simulink model "SimPIDlatdir2020b"  (R2020b)
settings: Solver=VariableStepAuto  StartTime=0.0  StopTime=10  RelTol=1e-3
values from neighbouring files (symbols this model uses):
  g_p_ail = tf(modelo(2,1))    [latdirPID.m]
  g_p_rud = tf(modelo(2,2))    [latdirPID.m]
  g_phi_ail = tf(modelo(4,1))    [latdirPID.m]
  g_phi_rud = tf(modelo(4,2))    [latdirPID.m]
  g_psi_ail = tf(modelo(5,2))    [latdirPID.m]
  g_psi_rud = tf(modelo(5,2))    [latdirPID.m]
  g_r_ail = tf(modelo(3,1))    [latdirPID.m]
  g_r_rud = tf(modelo(3,2))    [latdirPID.m]
  Kd_a = 2    [latdirPID.m]
  Kd_r = 2    [latdirPID.m]
  Ki_a = 0.002    [latdirPID.m]
  Ki_r = 0.002    [latdirPID.m]
  Kp_a = 7    [latdirPID.m]
  Kp_r = 7    [latdirPID.m]
libraries: pid_lib x16, simulink x4
(part 2 of 2)

== system SimPIDlatdir2020b/LatDir Ruido/Pos modelo/CAS_Yaw ==
  Ail : Inport
  Rud : Inport  Port=2
  CAS_ail : pid_lib/PID Controller  Controller=PI  Form=Parallel  TimeDomain=Continuous-time  UseExternalTs=off  SampleTime=-1  IntegratorMethod=Forward Euler  FilterMethod=Forward Euler  ControllerParametersSource=internal  P=Kp_a  I=Ki_a  D=0  N=100  UseFilter=on  TunerSelectOption=Transfer Function Based (PID Tuner App)  InitialConditionSource=internal  InitialConditionForIntegrator=0  InitialConditionForFilter=0  DifferentiatorICPrevScaledInput=0  ExternalReset=none  TrackingMode=off  Kt=1  LimitOutput=off  SatLimitsSource=internal  UpperSaturationLimit=inf  LowerSaturationLimit=-inf  LinearizeAsGain=on  AntiWindupMode=none  Kb=1  POutMin=[]  POutMax=[]  IOutMin=[]  IOutMax=[]  DOutMin=[]  DOutMax=[]  NOutMin=[]  NOutMax=[]  SumOutMin=[]  SumOutMax=[]  SaturationOutMin=[]  SaturationOutMax=[]  PParamMin=[]  PParamMax=[]  IParamMin=[]  IParamMax=[]  DParamMin=[]  DParamMax=[]  NParamMin=[]  NParamMax=[]  KbParamMin=[]  KbParamMax=[]  KtParamMin=[]  KtParamMax=[]  KbOutMin=[]  KbOutMax=[]  KtOutMin=[]  KtOutMax=[]  IntegratorOutMin=[]  IntegratorOutMax=[]  FilterOutMin=[]  FilterOutMax=[]  SumI1OutMin=[]  SumI1OutMax=[]  SumI2OutMin=[]  SumI2OutMax=[]  SumI3OutMin=[]  SumI3OutMax=[]  SumI4OutMin=[]  SumI4OutMax=[]  SumDOutMin=[]  SumDOutMax=[]  DifferentiatorOutMin=[]  DifferentiatorOutMax=[]  FilterDiffOutCoefMin=[]  FilterDiffOutCoefMax=[]  ReciprocalOutMin=[]  ReciprocalOutMax=[]  SumDenOutMin=[]  SumDenOutMax=[]  SumNumOutMin=[]  SumNumOutMax=[]  DivideOutMin=[]  DivideOutMax=[]  UdiffTsProdOutMin=[]  UdiffTsProdOutMax=[]  NTsProdOutMin=[]  NTsProdOutMax=[]  UintegralTsProdOutMin=[]  UintegralTsProdOutMax=[]  UngainTsProdOutMin=[]  UngainTsProdOutMax=[]  IntegratorContinuousStateAttributes=''  IntegratorStateMustResolveToSignalObject=off  IntegratorRTWStateStorageClass=Auto  FilterContinuousStateAttributes=''  FilterStateMustResolveToSignalObject=off  FilterRTWStateStorageClass=Auto  ParallelPVariant=InternalParameters  IdealPVariant=Disabled  IVariant=InternalParameters  DVariant=Disabled  IntegratorVariant=Continuous  SatVariant=Disabled  AWVariant=Passthrough  PCopyVariant=Disabled  TRVariant=Disabled  FdbkBlocksVariant=Forward  IdealPFdbkVariant=Disabled  SatFdbkVariant=Disabled  DerivativeFilterVariant=Disabled  NVariant=Disabled  NCopyVariant=Disabled_SignalSpec  FilterICVariant=Disabled  IntegratorICVariant=InternalICs  ExternalResetVariant=Disabled  TRSumVariant=Passthrough  SumFdbkVariant=Disabled  SumVariant=Sum_PI  TsampFilterVariant=InternalTs  TsampNgainVariant=Passthrough  TsampIntegralVariant=Passthrough  ExternalSaturationOutDataTypeStr=Inherit: Same as second input
  CAS_rud : pid_lib/PID Controller  Controller=PI  Form=Parallel  TimeDomain=Continuous-time  UseExternalTs=off  SampleTime=-1  IntegratorMethod=Forward Euler  FilterMethod=Forward Euler  ControllerParametersSource=internal  P=Kp_r  I=Ki_r  D=0  N=100  UseFilter=on  TunerSelectOption=Transfer Function Based (PID Tuner App)  InitialConditionSource=internal  InitialConditionForIntegrator=0  InitialConditionForFilter=0  DifferentiatorICPrevScaledInput=0  ExternalReset=none  TrackingMode=off  Kt=1  LimitOutput=off  SatLimitsSource=internal  UpperSaturationLimit=inf  LowerSaturationLimit=-inf  LinearizeAsGain=on  AntiWindupMode=none  Kb=1  POutMin=[]  POutMax=[]  IOutMin=[]  IOutMax=[]  DOutMin=[]  DOutMax=[]  NOutMin=[]  NOutMax=[]  SumOutMin=[]  SumOutMax=[]  SaturationOutMin=[]  SaturationOutMax=[]  PParamMin=[]  PParamMax=[]  IParamMin=[]  IParamMax=[]  DParamMin=[]  DParamMax=[]  NParamMin=[]  NParamMax=[]  KbParamMin=[]  KbParamMax=[]  KtParamMin=[]  KtParamMax=[]  KbOutMin=[]  KbOutMax=[]  KtOutMin=[]  KtOutMax=[]  IntegratorOutMin=[]  IntegratorOutMax=[]  FilterOutMin=[]  FilterOutMax=[]  SumI1OutMin=[]  SumI1OutMax=[]  SumI2OutMin=[]  SumI2OutMax=[]  SumI3OutMin=[]  SumI3OutMax=[]  SumI4OutMin=[]  SumI4OutMax=[]  SumDOutMin=[]  SumDOutMax=[]  DifferentiatorOutMin=[]  DifferentiatorOutMax=[]  FilterDiffOutCoefMin=[]  FilterDiffOutCoefMax=[]  ReciprocalOutMin=[]  ReciprocalOutMax=[]  SumDenOutMin=[]  SumDenOutMax=[]  SumNumOutMin=[]  SumNumOutMax=[]  DivideOutMin=[]  DivideOutMax=[]  UdiffTsProdOutMin=[]  UdiffTsProdOutMax=[]  NTsProdOutMin=[]  NTsProdOutMax=[]  UintegralTsProdOutMin=[]  UintegralTsProdOutMax=[]  UngainTsProdOutMin=[]  UngainTsProdOutMax=[]  IntegratorContinuousStateAttributes=''  IntegratorStateMustResolveToSignalObject=off  IntegratorRTWStateStorageClass=Auto  FilterContinuousStateAttributes=''  FilterStateMustResolveToSignalObject=off  FilterRTWStateStorageClass=Auto  ParallelPVariant=InternalParameters  IdealPVariant=Disabled  IVariant=InternalParameters  DVariant=Disabled  IntegratorVariant=Continuous  SatVariant=Disabled  AWVariant=Passthrough  PCopyVariant=Disabled  TRVariant=Disabled  FdbkBlocksVariant=Forward  IdealPFdbkVariant=Disabled  SatFdbkVariant=Disabled  DerivativeFilterVariant=Disabled  NVariant=Disabled  NCopyVariant=Disabled_SignalSpec  FilterICVariant=Disabled  IntegratorICVariant=InternalICs  ExternalResetVariant=Disabled  TRSumVariant=Passthrough  SumFdbkVariant=Disabled  SumVariant=Sum_PI  TsampFilterVariant=InternalTs  TsampNgainVariant=Passthrough  TsampIntegralVariant=Passthrough  ExternalSaturationOutDataTypeStr=Inherit: Same as second input
  SAS : Subsystem
  Sum : Sum  Inputs=-+|
  Sum1 : Sum  Inputs=|+-
  Psi : Outport
  wires:
  Sum1/1 -> CAS_rud/1
  Rud/1 -> Sum1/1
  Sum/1 -> CAS_ail/1
  CAS_rud/1 -> SAS/2("rud ")
  SAS/1(Psi) -> Psi/1, Sum1/2, Sum/1
  CAS_ail/1 -> SAS/1(ail)
  Ail/1 -> Sum/2

== system SimPIDlatdir2020b/LatDir/Pos integrada/CAS_Roll2/SAS ==
  note: Se realimenta la velocidad del ángulo phi como contribución de
      | cada uno de los actuadores.
  ail : Inport
  "rud " : Inport  Port=2
  Kd_ail : Gain  Gain=Kd_a
  Kd_rud : Gain  Gain=Kd_r
  Roll : Subsystem
  Sum : Sum  Inputs=-+|
  Sum1 : Sum  Inputs=|+-
  Phi : Outport
  wires:
  Sum1/1 -> Roll/2("rud ")
  Sum/1 -> Roll/1(ail)
  Kd_rud/1 -> Sum1/2
  Kd_ail/1 -> Sum/1
  ail/1 -> Sum/2
  "rud "/1 -> Sum1/1
  Roll/1(Phi) -> Phi/1
  Roll/2(Phi_dot) -> Kd_ail/1, Kd_rud/1

== system SimPIDlatdir2020b/LatDir/Pos integrada/CAS_Yaw2/SAS ==
  note: Se realimenta la velocidad del ángulo phi como contribución de
      | cada uno de los actuadores.
  ail : Inport
  "rud " : Inport  Port=2
  Kd_ail : Gain  Gain=Kd_a
  Kd_rud : Gain  Gain=Kd_r
  Sum : Sum  Inputs=-+|
  Sum1 : Sum  Inputs=|+-
  Yaw : Subsystem
  Psi : Outport
  wires:
  Yaw/2(Psi_dot) -> Kd_ail/1, Kd_rud/1
  Yaw/1(Psi) -> Psi/1
  "rud "/1 -> Sum1/1
  ail/1 -> Sum/2
  Kd_ail/1 -> Sum/1
  Kd_rud/1 -> Sum1/2
  Sum/1 -> Yaw/1(ail)
  Sum1/1 -> Yaw/2("rud ")

== system SimPIDlatdir2020b/LatDir/Pos modelo/CAS_Roll/SAS ==
  note: Se realimenta la velocidad del ángulo phi como contribución de
      | cada uno de los actuadores.
  ail : Inport
  "rud " : Inport  Port=2
  Kd_ail : Gain  Gain=Kd_a
  Kd_rud : Gain  Gain=Kd_r
  Roll : Subsystem
  Sum : Sum  Inputs=-+|
  Sum1 : Sum  Inputs=|+-
  Phi : Outport
  wires:
  Roll/2(Phi_dot) -> Kd_rud/1, Kd_ail/1
  Roll/1(Phi) -> Phi/1
  "rud "/1 -> Sum1/1
  ail/1 -> Sum/2
  Kd_ail/1 -> Sum/1
  Kd_rud/1 -> Sum1/2
  Sum/1 -> Roll/1(ail)
  Sum1/1 -> Roll/2("rud ")

== system SimPIDlatdir2020b/LatDir/Pos modelo/CAS_Yaw/SAS ==
  note: Se realimenta la velocidad del ángulo phi como contribución de
      | cada uno de los actuadores.
  ail : Inport
  "rud " : Inport  Port=2
  Kd_ail : Gain  Gain=Kd_a
  Kd_rud : Gain  Gain=Kd_r
  Sum : Sum  Inputs=-+|
  Sum1 : Sum  Inputs=|+-
  Yaw : Subsystem
  Psi : Outport
  wires:
  Sum1/1 -> Yaw/2("rud ")
  Sum/1 -> Yaw/1(ail)
  Kd_rud/1 -> Sum1/2
  Kd_ail/1 -> Sum/1
  ail/1 -> Sum/2
  "rud "/1 -> Sum1/1
  Yaw/1(Psi) -> Psi/1
  Yaw/2(Psi_dot) -> Kd_rud/1, Kd_ail/1

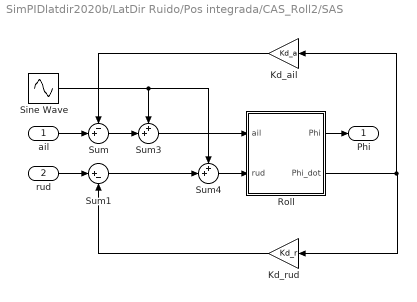
== system SimPIDlatdir2020b/LatDir Ruido/Pos integrada/CAS_Roll2/SAS ==
  ail : Inport
  "rud " : Inport  Port=2
  Kd_ail : Gain  Gain=Kd_a
  Kd_rud : Gain  Gain=Kd_r
  Roll : Subsystem
  Sine Wave : Sin  SampleTime=0
  Sum : Sum  Inputs=-+|
  Sum1 : Sum  Inputs=|+-
  Sum3 : Sum  Inputs=++|
  Sum4 : Sum  Inputs=++|
  Phi : Outport
  wires:
  Roll/1(Phi) -> Phi/1
  "rud "/1 -> Sum1/1
  ail/1 -> Sum/2
  Kd_ail/1 -> Sum/1
  Kd_rud/1 -> Sum1/2
  Sum1/1 -> Sum4/2
  Sum4/1 -> Roll/2("rud ")
  Sum/1 -> Sum3/2
  Sum3/1 -> Roll/1(ail)
  Sine Wave/1 -> Sum4/1, Sum3/1
  Roll/2(Phi_dot) -> Kd_ail/1, Kd_rud/1

== system SimPIDlatdir2020b/LatDir Ruido/Pos integrada/CAS_Yaw2/SAS ==
  ail : Inport
  "rud " : Inport  Port=2
  Kd_ail : Gain  Gain=Kd_a
  Kd_rud : Gain  Gain=Kd_r
  Sum : Sum  Inputs=-+|
  Sum1 : Sum  Inputs=|+-
  Yaw : Subsystem
  Psi : Outport
  wires:
  Sum1/1 -> Yaw/2("rud ")
  Sum/1 -> Yaw/1(ail)
  Kd_rud/1 -> Sum1/2
  Kd_ail/1 -> Sum/1
  ail/1 -> Sum/2
  "rud "/1 -> Sum1/1
  Yaw/1(Psi) -> Psi/1
  Yaw/2(Psi_dot) -> Kd_rud/1, Kd_ail/1

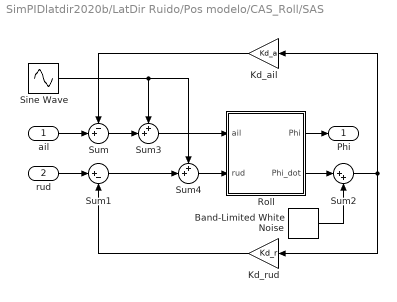
== system SimPIDlatdir2020b/LatDir Ruido/Pos modelo/CAS_Roll/SAS ==
  ail : Inport
  "rud " : Inport  Port=2
  Band-Limited White Noise : simulink/Sources/Band-Limited White Noise  Cov=[0.001]  Ts=0.1  seed=[23341]
  Kd_ail : Gain  Gain=Kd_a
  Kd_rud : Gain  Gain=Kd_r
  Roll : Subsystem
  Sine Wave : Sin  Frequency=12*pi  SampleTime=0
  Sum : Sum  Inputs=-+|
  Sum1 : Sum  Inputs=|+-
  Sum2 : Sum  Inputs=|++
  Sum3 : Sum  Inputs=++|
  Sum4 : Sum  Inputs=++|
  Phi : Outport
  wires:
  Kd_rud/1 -> Sum1/2
  Kd_ail/1 -> Sum/1
  ail/1 -> Sum/2
  "rud "/1 -> Sum1/1
  Roll/1(Phi) -> Phi/1
  Roll/2(Phi_dot) -> Sum2/1
  Sum2/1 -> Kd_rud/1, Kd_ail/1
  Band-Limited White Noise/1 -> Sum2/2
  Sum/1 -> Sum3/2
  Sum3/1 -> Roll/1(ail)
  Sum4/1 -> Roll/2("rud ")
  Sum1/1 -> Sum4/2
  Sine Wave/1 -> Sum4/1, Sum3/1

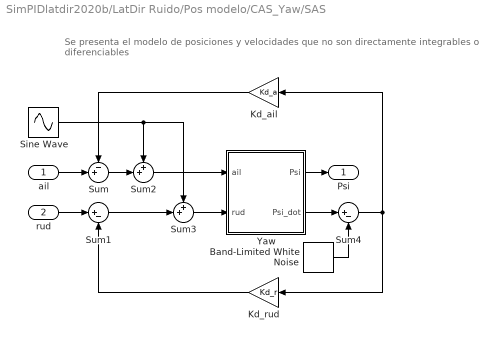
== system SimPIDlatdir2020b/LatDir Ruido/Pos modelo/CAS_Yaw/SAS ==
  note: Se presenta el modelo de posiciones y velocidades que no son directamente integrables o diferenciables
  ail : Inport
  "rud " : Inport  Port=2
  Band-Limited White Noise : simulink/Sources/Band-Limited White Noise  Cov=0.001  Ts=0.1  seed=[23341]
  Kd_ail : Gain  Gain=Kd_a
  Kd_rud : Gain  Gain=Kd_r
  Sine Wave : Sin  Frequency=12*pi  SampleTime=0
  Sum : Sum  Inputs=-+|
  Sum1 : Sum  Inputs=|+-
  Sum2 : Sum  Inputs=++|
  Sum3 : Sum  Inputs=++|
  Sum4 : Sum  Inputs=|+-
  Yaw : Subsystem
  Psi : Outport
  wires:
  Yaw/1(Psi) -> Psi/1
  "rud "/1 -> Sum1/1
  ail/1 -> Sum/2
  Kd_ail/1 -> Sum/1
  Kd_rud/1 -> Sum1/2
  Sum/1 -> Sum2/2
  Sum2/1 -> Yaw/1(ail)
  Sum3/1 -> Yaw/2("rud ")
  Sum1/1 -> Sum3/2
  Sine Wave/1 -> Sum3/1, Sum2/1
  Yaw/2(Psi_dot) -> Sum4/1
  Sum4/1 -> Kd_ail/1, Kd_rud/1
  Band-Limited White Noise/1 -> Sum4/2

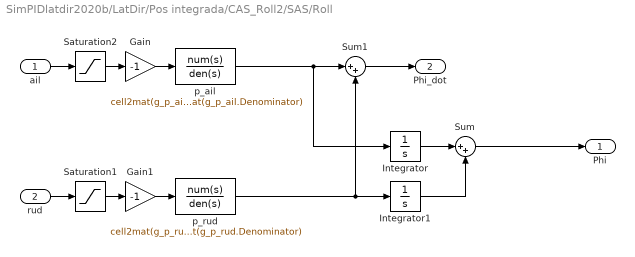
== system SimPIDlatdir2020b/LatDir/Pos integrada/CAS_Roll2/SAS/Roll ==
  ail : Inport
  "rud " : Inport  Port=2
  Gain : Gain  Gain=-1
  Gain1 : Gain  Gain=-1
  Integrator : Integrator
  Integrator1 : Integrator
  Saturation1 : Saturate  UpperLimit=30  LowerLimit=-30
  Saturation2 : Saturate  UpperLimit=30  LowerLimit=-30
  Sum : Sum  Inputs=|++
  Sum1 : Sum  Inputs=|++
  p_ail : TransferFcn  Numerator=cell2mat(g_p_ail.Numerator)  Denominator=cell2mat(g_p_ail.Denominator)
  p_rud : TransferFcn  Numerator=cell2mat(g_p_rud.Numerator)  Denominator=cell2mat(g_p_rud.Denominator)
  Phi : Outport
  Phi_dot : Outport  Port=2
  wires:
  "rud "/1 -> Saturation1/1
  Gain1/1 -> p_rud/1
  Gain/1 -> p_ail/1
  Sum/1 -> Phi/1
  Sum1/1 -> Phi_dot/1
  p_ail/1 -> Integrator/1, Sum1/1
  p_rud/1 -> Sum1/2, Integrator1/1
  ail/1 -> Saturation2/1
  Integrator/1 -> Sum/1
  Integrator1/1 -> Sum/2
  Saturation2/1 -> Gain/1
  Saturation1/1 -> Gain1/1

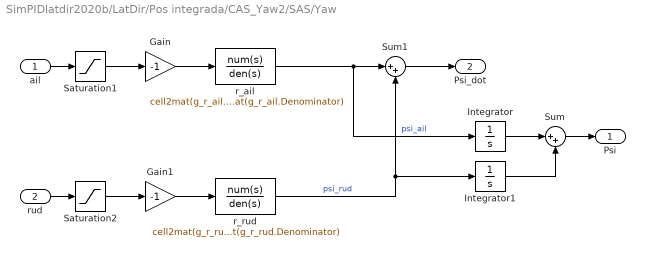
== system SimPIDlatdir2020b/LatDir/Pos integrada/CAS_Yaw2/SAS/Yaw ==
  ail : Inport
  "rud " : Inport  Port=2
  Gain : Gain  Gain=-1
  Gain1 : Gain  Gain=-1
  Integrator : Integrator
  Integrator1 : Integrator
  Saturation1 : Saturate  UpperLimit=30  LowerLimit=-30
  Saturation2 : Saturate  UpperLimit=30  LowerLimit=-30
  Sum : Sum  Inputs=|++
  Sum1 : Sum  Inputs=|++
  r_ail : TransferFcn  Numerator=cell2mat(g_r_ail.Numerator)  Denominator=cell2mat(g_r_ail.Denominator)
  r_rud : TransferFcn  Numerator=cell2mat(g_r_rud.Numerator)  Denominator=cell2mat(g_r_rud.Denominator)
  Psi : Outport
  Psi_dot : Outport  Port=2
  wires:
  "rud "/1 -> Saturation2/1
  ail/1 -> Saturation1/1
  r_rud/1 -> Integrator1/1, Sum1/2  "psi_rud"
  r_ail/1 -> Integrator/1, Sum1/1  "psi_ail"
  Sum1/1 -> Psi_dot/1
  Sum/1 -> Psi/1
  Integrator1/1 -> Sum/2
  Integrator/1 -> Sum/1
  Saturation1/1 -> Gain/1
  Saturation2/1 -> Gain1/1
  Gain/1 -> r_ail/1
  Gain1/1 -> r_rud/1

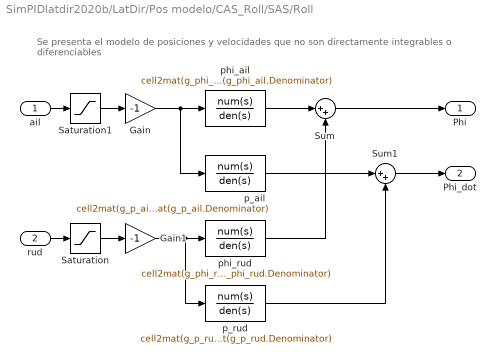
== system SimPIDlatdir2020b/LatDir/Pos modelo/CAS_Roll/SAS/Roll ==
  note: Se presenta el modelo de posiciones y velocidades que no son directamente integrables o diferenciables
  ail : Inport
  "rud " : Inport  Port=2
  Gain : Gain  Gain=-1
  Gain1 : Gain  Gain=-1
  Saturation : Saturate  UpperLimit=30  LowerLimit=-30
  Saturation1 : Saturate  UpperLimit=30  LowerLimit=-30
  Sum : Sum  Inputs=|++
  Sum1 : Sum  Inputs=|++
  p_ail : TransferFcn  Numerator=cell2mat(g_p_ail.Numerator)  Denominator=cell2mat(g_p_ail.Denominator)
  p_rud : TransferFcn  Numerator=cell2mat(g_p_rud.Numerator)  Denominator=cell2mat(g_p_rud.Denominator)
  phi_ail : TransferFcn  Numerator=cell2mat(g_phi_ail.Numerator)  Denominator=cell2mat(g_phi_ail.Denominator)
  phi_rud : TransferFcn  Numerator=cell2mat(g_phi_rud.Numerator)  Denominator=cell2mat(g_phi_rud.Denominator)
  Phi : Outport
  Phi_dot : Outport  Port=2
  wires:
  ail/1 -> Saturation1/1
  p_rud/1 -> Sum1/2
  p_ail/1 -> Sum1/1
  phi_ail/1 -> Sum/1
  Sum1/1 -> Phi_dot/1
  phi_rud/1 -> Sum/2
  Sum/1 -> Phi/1
  Gain/1 -> p_ail/1, phi_ail/1
  Gain1/1 -> p_rud/1, phi_rud/1
  "rud "/1 -> Saturation/1
  Saturation/1 -> Gain1/1
  Saturation1/1 -> Gain/1

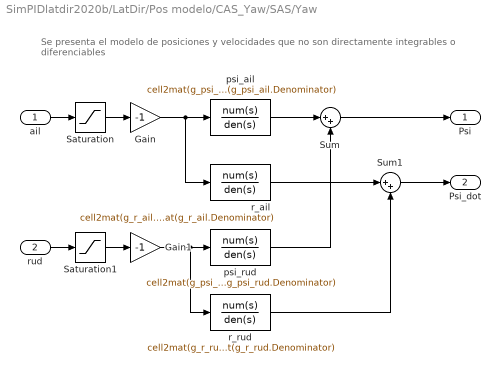
== system SimPIDlatdir2020b/LatDir/Pos modelo/CAS_Yaw/SAS/Yaw ==
  note: Se presenta el modelo de posiciones y velocidades que no son directamente integrables o diferenciables
  ail : Inport
  "rud " : Inport  Port=2
  Gain : Gain  Gain=-1
  Gain1 : Gain  Gain=-1
  Saturation : Saturate  UpperLimit=30  LowerLimit=-30
  Saturation1 : Saturate  UpperLimit=30  LowerLimit=-30
  Sum : Sum  Inputs=|++
  Sum1 : Sum  Inputs=|++
  psi_ail : TransferFcn  Numerator=cell2mat(g_psi_ail.Numerator)  Denominator=cell2mat(g_psi_ail.Denominator)
  psi_rud : TransferFcn  Numerator=cell2mat(g_psi_rud.Numerator)  Denominator=cell2mat(g_psi_rud.Denominator)
  r_ail : TransferFcn  Numerator=cell2mat(g_r_ail.Numerator)  Denominator=cell2mat(g_r_ail.Denominator)
  r_rud : TransferFcn  Numerator=cell2mat(g_r_rud.Numerator)  Denominator=cell2mat(g_r_rud.Denominator)
  Psi : Outport
  Psi_dot : Outport  Port=2
  wires:
  Sum/1 -> Psi/1
  psi_rud/1 -> Sum/2
  Sum1/1 -> Psi_dot/1
  psi_ail/1 -> Sum/1
  r_ail/1 -> Sum1/1
  r_rud/1 -> Sum1/2
  ail/1 -> Saturation/1
  "rud "/1 -> Saturation1/1
  Gain/1 -> r_ail/1, psi_ail/1
  Gain1/1 -> r_rud/1, psi_rud/1
  Saturation/1 -> Gain/1
  Saturation1/1 -> Gain1/1

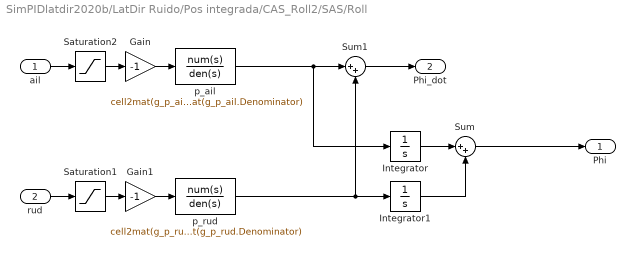
== system SimPIDlatdir2020b/LatDir Ruido/Pos integrada/CAS_Roll2/SAS/Roll ==
  ail : Inport
  "rud " : Inport  Port=2
  Gain : Gain  Gain=-1
  Gain1 : Gain  Gain=-1
  Integrator : Integrator
  Integrator1 : Integrator
  Saturation1 : Saturate  UpperLimit=30  LowerLimit=-30
  Saturation2 : Saturate  UpperLimit=30  LowerLimit=-30
  Sum : Sum  Inputs=|++
  Sum1 : Sum  Inputs=|++
  p_ail : TransferFcn  Numerator=cell2mat(g_p_ail.Numerator)  Denominator=cell2mat(g_p_ail.Denominator)
  p_rud : TransferFcn  Numerator=cell2mat(g_p_rud.Numerator)  Denominator=cell2mat(g_p_rud.Denominator)
  Phi : Outport
  Phi_dot : Outport  Port=2
  wires:
  Saturation1/1 -> Gain1/1
  Saturation2/1 -> Gain/1
  Integrator1/1 -> Sum/2
  Integrator/1 -> Sum/1
  ail/1 -> Saturation2/1
  p_rud/1 -> Integrator1/1, Sum1/2
  p_ail/1 -> Sum1/1, Integrator/1
  Sum1/1 -> Phi_dot/1
  Sum/1 -> Phi/1
  Gain/1 -> p_ail/1
  Gain1/1 -> p_rud/1
  "rud "/1 -> Saturation1/1

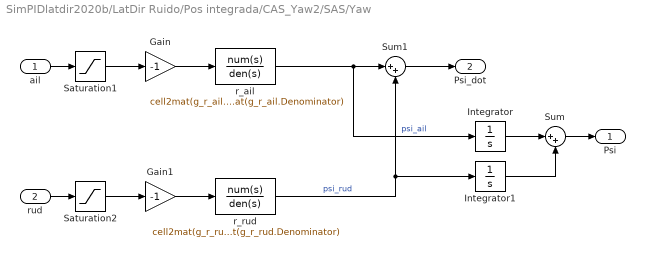
== system SimPIDlatdir2020b/LatDir Ruido/Pos integrada/CAS_Yaw2/SAS/Yaw ==
  ail : Inport
  "rud " : Inport  Port=2
  Gain : Gain  Gain=-1
  Gain1 : Gain  Gain=-1
  Integrator : Integrator
  Integrator1 : Integrator
  Saturation1 : Saturate  UpperLimit=30  LowerLimit=-30
  Saturation2 : Saturate  UpperLimit=30  LowerLimit=-30
  Sum : Sum  Inputs=|++
  Sum1 : Sum  Inputs=|++
  r_ail : TransferFcn  Numerator=cell2mat(g_r_ail.Numerator)  Denominator=cell2mat(g_r_ail.Denominator)
  r_rud : TransferFcn  Numerator=cell2mat(g_r_rud.Numerator)  Denominator=cell2mat(g_r_rud.Denominator)
  Psi : Outport
  Psi_dot : Outport  Port=2
  wires:
  Gain1/1 -> r_rud/1
  Gain/1 -> r_ail/1
  Saturation2/1 -> Gain1/1
  Saturation1/1 -> Gain/1
  Integrator/1 -> Sum/1
  Integrator1/1 -> Sum/2
  Sum/1 -> Psi/1
  Sum1/1 -> Psi_dot/1
  r_ail/1 -> Sum1/1, Integrator/1  "psi_ail"
  r_rud/1 -> Sum1/2, Integrator1/1  "psi_rud"
  ail/1 -> Saturation1/1
  "rud "/1 -> Saturation2/1

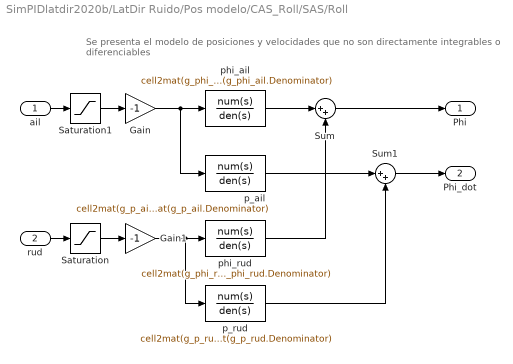
== system SimPIDlatdir2020b/LatDir Ruido/Pos modelo/CAS_Roll/SAS/Roll ==
  note: Se presenta el modelo de posiciones y velocidades que no son directamente integrables o diferenciables
  ail : Inport
  "rud " : Inport  Port=2
  Gain : Gain  Gain=-1
  Gain1 : Gain  Gain=-1
  Saturation : Saturate  UpperLimit=30  LowerLimit=-30
  Saturation1 : Saturate  UpperLimit=30  LowerLimit=-30
  Sum : Sum  Inputs=|++
  Sum1 : Sum  Inputs=|++
  p_ail : TransferFcn  Numerator=cell2mat(g_p_ail.Numerator)  Denominator=cell2mat(g_p_ail.Denominator)
  p_rud : TransferFcn  Numerator=cell2mat(g_p_rud.Numerator)  Denominator=cell2mat(g_p_rud.Denominator)
  phi_ail : TransferFcn  Numerator=cell2mat(g_phi_ail.Numerator)  Denominator=cell2mat(g_phi_ail.Denominator)
  phi_rud : TransferFcn  Numerator=cell2mat(g_phi_rud.Numerator)  Denominator=cell2mat(g_phi_rud.Denominator)
  Phi : Outport
  Phi_dot : Outport  Port=2
  wires:
  Saturation1/1 -> Gain/1
  Saturation/1 -> Gain1/1
  "rud "/1 -> Saturation/1
  Gain1/1 -> phi_rud/1, p_rud/1
  Gain/1 -> phi_ail/1, p_ail/1
  Sum/1 -> Phi/1
  phi_rud/1 -> Sum/2
  Sum1/1 -> Phi_dot/1
  phi_ail/1 -> Sum/1
  p_ail/1 -> Sum1/1
  p_rud/1 -> Sum1/2
  ail/1 -> Saturation1/1

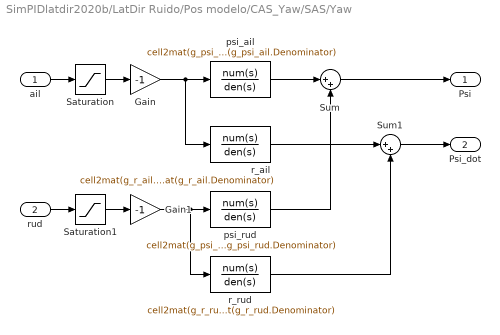
== system SimPIDlatdir2020b/LatDir Ruido/Pos modelo/CAS_Yaw/SAS/Yaw ==
  ail : Inport
  "rud " : Inport  Port=2
  Gain : Gain  Gain=-1
  Gain1 : Gain  Gain=-1
  Saturation : Saturate  UpperLimit=30  LowerLimit=-30
  Saturation1 : Saturate  UpperLimit=30  LowerLimit=-30
  Sum : Sum  Inputs=|++
  Sum1 : Sum  Inputs=|++
  psi_ail : TransferFcn  Numerator=cell2mat(g_psi_ail.Numerator)  Denominator=cell2mat(g_psi_ail.Denominator)
  psi_rud : TransferFcn  Numerator=cell2mat(g_psi_rud.Numerator)  Denominator=cell2mat(g_psi_rud.Denominator)
  r_ail : TransferFcn  Numerator=cell2mat(g_r_ail.Numerator)  Denominator=cell2mat(g_r_ail.Denominator)
  r_rud : TransferFcn  Numerator=cell2mat(g_r_rud.Numerator)  Denominator=cell2mat(g_r_rud.Denominator)
  Psi : Outport
  Psi_dot : Outport  Port=2
  wires:
  Saturation1/1 -> Gain1/1
  Saturation/1 -> Gain/1
  Gain1/1 -> psi_rud/1, r_rud/1
  Gain/1 -> psi_ail/1, r_ail/1
  "rud "/1 -> Saturation1/1
  ail/1 -> Saturation/1
  r_rud/1 -> Sum1/2
  r_ail/1 -> Sum1/1
  psi_ail/1 -> Sum/1
  Sum1/1 -> Psi_dot/1
  psi_rud/1 -> Sum/2
  Sum/1 -> Psi/1
